simulink model "EV3_MatSys_Demo_WiFI"  (R2023a)
settings: Solver=FixedStepAuto  StartTime=0.0  StopTime=10.0  FixedStep=0.1  RelTol=1e-3
libraries: realtime_pacer_lib x1
settings Model: Creator=chris  LastModifiedBy=Christian

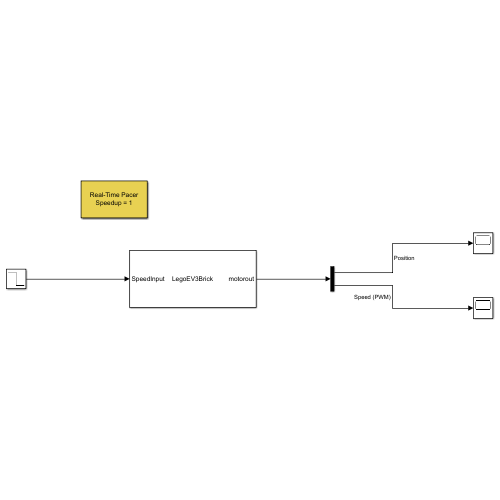
[thumbnail: Simulink's stored preview of the top-level diagram]
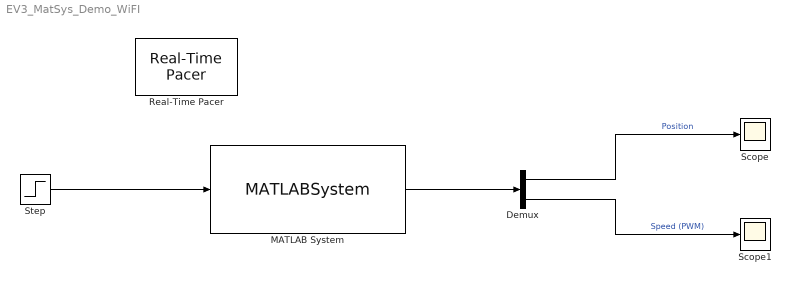
== system EV3_MatSys_Demo_WiFI ==
  Demux : Demux  Outputs=2
  MATLAB System : MATLABSystem  System=LegoEV3Brick  address=192.168.87.151  motorport=A  id=0016534cde97  SimulateUsing=Interpreted execution
      mask Type: LegoEV3Brick
      mask Display:
      | disp('LegoEV3Brick');
      | port_label('input',1,'SpeedInput');
      | port_label('output',1,'motorout');
  Real-Time Pacer : realtime_pacer_lib/Real-Time Pacer  simTimePerRealTime=1
  Scope : Scope
  Scope1 : Scope
  Step : Step  Time=5  Before=100  After=-100
  wires:
  MATLAB System/1 -> Demux/1
  Step/1 -> MATLAB System/1
  Demux/1 -> Scope/1  "Position"
  Demux/2 -> Scope1/1  "Speed (PWM)"
